simulink model "ex2_simulare_rasp_met2"  (R2020a)
settings: Solver=VariableStepAuto  StartTime=0.0  StopTime=10.0  RelTol=1e-3

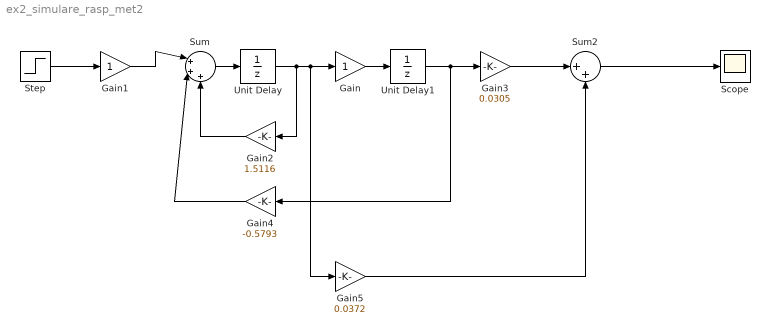
== system ex2_simulare_rasp_met2 ==
  Gain : Gain
  Gain1 : Gain
  Gain2 : Gain  Gain=1.5116
  Gain3 : Gain  Gain=0.0305
  Gain4 : Gain  Gain=-0.5793
  Gain5 : Gain  Gain=0.0372
  Scope : Scope
  Step : Step  SampleTime=0.1
  Sum : Sum  Inputs=|+++
  Sum2 : Sum  Inputs=|++
  Unit Delay : UnitDelay  SampleTime=-1  HasFrameUpgradeWarning=on
  Unit Delay1 : UnitDelay  SampleTime=-1  HasFrameUpgradeWarning=on
  wires:
  Step/1 -> Gain1/1
  Sum/1 -> Unit Delay/1
  Unit Delay/1 -> Gain/1, Gain5/1, Gain2/1
  Gain/1 -> Unit Delay1/1
  Unit Delay1/1 -> Gain3/1, Gain4/1
  Gain1/1 -> Sum/1
  Gain2/1 -> Sum/3
  Gain4/1 -> Sum/2
  Sum2/1 -> Scope/1
  Gain5/1 -> Sum2/2
  Gain3/1 -> Sum2/1
